simulink model "real_LAB3_PID"  (R2025b)
settings: Solver=ode3  StartTime=0.0  StopTime=10  FixedStep=0.001  RelTol=1e-3
values from neighbouring files (symbols this model uses):
  Kd = Kp * Td    [LAB3_design_controller.m]
  Ki = Kp / Ti    [LAB3_design_controller.m]
  Kp = Delta_K * cos(Delta_phi)    [LAB3_design_controller.m]
  Kw = 0    [diScorta.m]    (also in real_LAB3.m; sim_LAB3.m = 5.88235294118)
  step_amplitude = 50    [diScorta.m]    (also in real_LAB3.m)
  Tl = 1 / (10 * w_n)    [diScorta.m]    (also in real_LAB3.m; sim_LAB3.m)
  Ts = 0.001    [diScorta.m]    (also in real_LAB3.m; real_estimation.m; sim_LAB3.m)
undefined symbols (not defined in the file or in its folder): National_Instruments, PCI, sens
libraries: sldrtlib x2
settings Model: SimulationMode=external  ExtModeTrigDuration=100001  Creator=delpratogi  LastModifiedBy=ester
settings DataIOCC: ReturnWorkspaceOutputs=off
settings HardwareCC: ProdBitPerLong=64.0  ProdHWDeviceType=Intel->x86-64 (Linux 64)
settings RTWCC: SystemTargetFile=sldrt.tlc  TemplateMakefile=sldrt.tmf  RTWCompilerOptimization=on  Description=Simulink Desktop Real-Time
settings CodeAppCC: MaxIdLength=95.0
settings SimulinkDesktopRealTimeCC: ExtModeTransport=0.0  ExtModeStaticAllocSize=1000000.0  TargetLibSuffix=_sldrt.a  TargetPreCompLibLocation=C:\Program Files\MATLAB\R2025b\toolbox\sldrt\lib\win64  MultiwordLength=2048.0  DynamicStringBufferSize=256.0  ParMdlRefBuildCompliant=on  PreserveMATLABNamespacesInGeneratedCode=on  SubcomponentCodeInterfacePackaging=Reusable function

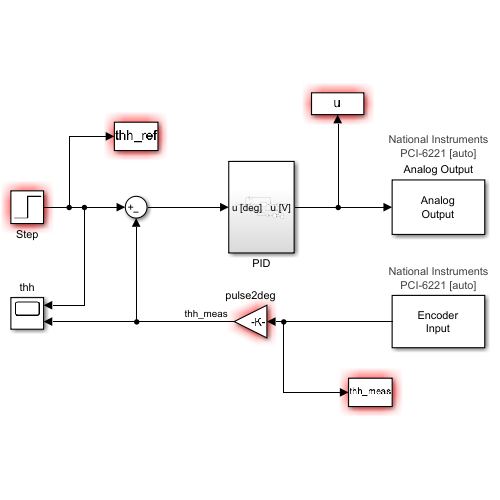
[thumbnail: Simulink's stored preview of the top-level diagram]
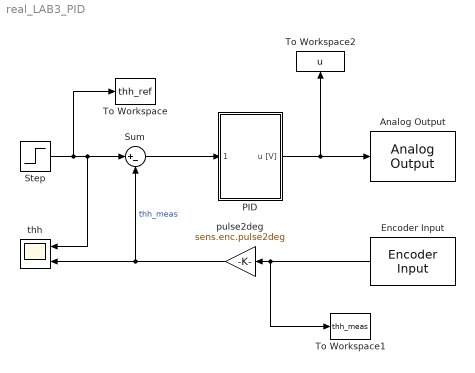
== system real_LAB3_PID ==
  Analog Output : sldrtlib/Analog Output  SampleTime=0.001  MaxMissedTicks=10  ShowMissedTicks=off  YieldWhenWaiting=off  DrvName=National_Instruments/PCI-6221  DrvAddress=4294967295  DrvOptions=[0 0 0 2 0]  Channels=1  RangeMode=1  VoltRange=1  InitialValue=0  FinalValue=0
      settings: AttributesFormatString=National Instruments\nPCI-6221 [auto]
  Encoder Input : sldrtlib/Encoder Input  SampleTime=0.001  MaxMissedTicks=10  ShowMissedTicks=off  YieldWhenWaiting=off  DrvName=National_Instruments/PCI-6221  DrvAddress=4294967295  DrvOptions=[0 0 0 2 0]  Channels=1  QuadMode=3  IndexPulse=1  InputFilter=Inf  DataType=1
      settings: AttributesFormatString=National Instruments\nPCI-6221 [auto]
  PID : Subsystem
  Step : Step  After=step_amplitude  SampleTime=Ts
  Sum : Sum  Inputs=|+-
  To Workspace : ToWorkspace  VariableName=thh_ref  SaveFormat=Structure With Time  SampleTime=Ts
  To Workspace1 : ToWorkspace  VariableName=thh_meas  SaveFormat=Structure With Time  SampleTime=Ts
  To Workspace2 : ToWorkspace  VariableName=u  SaveFormat=Structure With Time  SampleTime=Ts
  pulse2deg : Gain  Gain=sens.enc.pulse2deg
  thh : Scope  NumInputPorts=2
      settings: ActiveDisplayYMinimum=-6.2503462089638822  ActiveDisplayYMaximum=56.250038467662655
  wires:
  pulse2deg/1 -> Sum/2, thh/2  "thh_meas"
  Step/1 -> To Workspace/1, thh/1, Sum/1
  Sum/1 -> PID/1(u [deg])
  Encoder Input/1 -> To Workspace1/1, pulse2deg/1
  PID/1(u [V]) -> Analog Output/1, To Workspace2/1

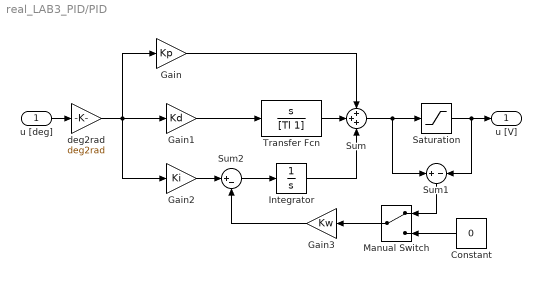
== system real_LAB3_PID/PID ==
  u [deg] : Inport
  Constant : Constant  Value=0
  Gain : Gain  Gain=Kp
  Gain1 : Gain  Gain=Kd
  Gain2 : Gain  Gain=Ki
  Gain3 : Gain  Gain=Kw
  Integrator : Integrator
  Manual Switch : ManualSwitch
  Saturation : Saturate  UpperLimit=10  LowerLimit=-10
  Sum : Sum  Inputs=+++
  Sum1 : Sum  Inputs=+-
  Sum2 : Sum  Inputs=|+-
  Transfer Fcn : TransferFcn  Numerator=[1 0]  Denominator=[Tl 1]
  deg2rad : Gain  Gain=deg2rad
  u [V] : Outport
  wires:
  Integrator/1 -> Sum/3
  Gain1/1 -> Transfer Fcn/1
  Gain/1 -> Sum/1
  Transfer Fcn/1 -> Sum/2
  u [deg]/1 -> deg2rad/1
  Sum/1 -> Saturation/1, Sum1/1
  Sum1/1 -> Manual Switch/1
  Saturation/1 -> Sum1/2, u [V]/1
  Manual Switch/1 -> Gain3/1
  Constant/1 -> Manual Switch/2
  Gain2/1 -> Sum2/1
  Sum2/1 -> Integrator/1
  Gain3/1 -> Sum2/2
  deg2rad/1 -> Gain2/1, Gain1/1, Gain/1
